simulink model "QPSK_system_v3e"  (R2012b)
settings: Solver=FixedStepDiscrete  SolverMode=SingleTasking  StartTime=0.0  StopTime=6000  FixedStep=1  RelTol=1e-3
libraries: simulink x30, dspsigops x2, dspbuff3 x1, dspsrcs4 x1
(part 1 of 4)
settings Model: FPTRunName=FPA_Reference  Creator=Carl  LastModifiedBy=castone
settings DataIOCC: SignalLogging=off
settings OptimizationCC: BlockReduction=off  ConditionallyExecuteInputs=off  InlineParams=on
settings DebuggingCC: AlgebraicLoopMsg=error
settings HardwareCC: ProdHWDeviceType=ASIC/FPGA->ASIC/FPGA  ProdEqTarget=off

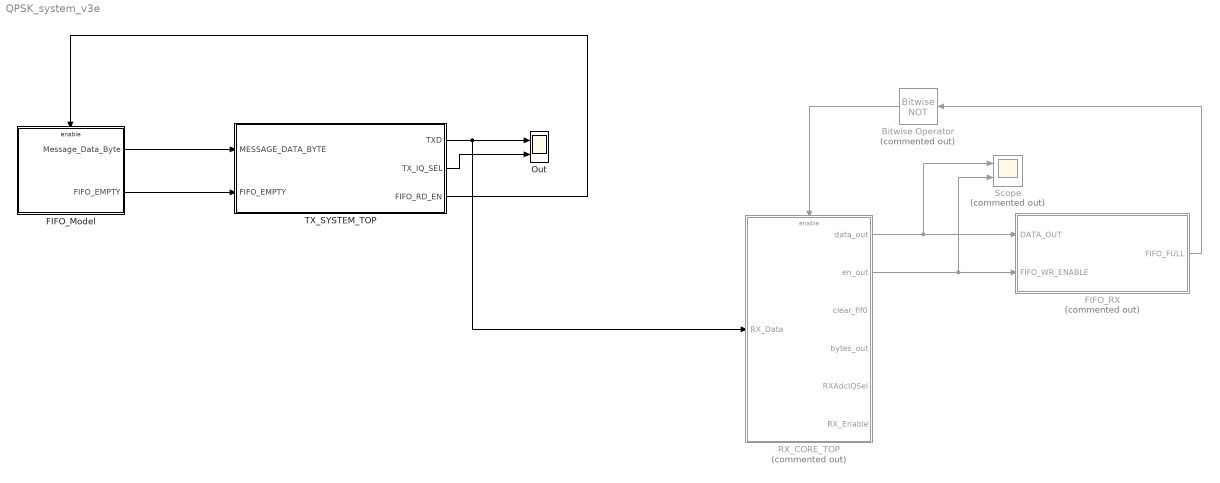
== system QPSK_system_v3e ==
  Bitwise Operator : simulink/Logic and Bit Operations/Bitwise Operator  Commented=on  logicop=NOT  UseBitMask=off  BitMask=bin2dec('11011001')  BitMaskRealWorld=Stored Integer
  FIFO_Model : Subsystem
  FIFO_RX : Subsystem  Commented=on
  Out : Scope  NumInputPorts=2
      settings: YMin=-5~-5  YMax=5~5  SaveName=ScopeData7
  RX_CORE_TOP : Subsystem  Commented=on
  Scope : Scope  Commented=on  NumInputPorts=2
      settings: YMin=-5~-5  YMax=5~5  SaveName=ScopeData20
  TX_SYSTEM_TOP : Subsystem
  wires:
  FIFO_Model/1(Message_Data_Byte) -> TX_SYSTEM_TOP/1(MESSAGE_DATA_BYTE)
  FIFO_Model/2(FIFO_EMPTY) -> TX_SYSTEM_TOP/2(FIFO_EMPTY)
  TX_SYSTEM_TOP/3(FIFO_RD_EN) -> FIFO_Model/Enable
  TX_SYSTEM_TOP/1(TXD) -> RX_CORE_TOP/1(RX_Data), Out/1
  TX_SYSTEM_TOP/2(TX_IQ_SEL) -> Out/2
  RX_CORE_TOP/1(data_out) -> FIFO_RX/1(DATA_OUT), Scope/1
  RX_CORE_TOP/2(en_out) -> FIFO_RX/2(FIFO_WR_ENABLE), Scope/2
  Bitwise Operator/1 -> RX_CORE_TOP/Enable
  FIFO_RX/1(FIFO_FULL) -> Bitwise Operator/1

== system QPSK_system_v3e/FIFO_Model ==
  Enable : EnablePort
  Compare To Constant5 : simulink/Logic and Bit Operations/Compare To Constant  relop===  const=17  OutDataTypeStr=boolean  ZeroCross=off
  Delay : Delay  DelayLength=1  InitialCondition=0
  Message_Data_LUT : LookupNDDirect  NumberOfTableDimensions=1  Table="[12        0        0        1        104        101        108        108        111        32        119        111        114        108        100        33        198        228]"  DiagnosticForOutOfRangeInput=Error  TableDataTypeStr=uint8
  Scope : Scope
  reset_counter : Subsystem  AncestorBlock=hdldemolib/HDL Streaming FFT/enable_counter
  Message_Data_Byte : Outport
  FIFO_EMPTY : Outport  Port=2
  wires:
  Message_Data_LUT/1 -> Message_Data_Byte/1
  reset_counter/1(sclock) -> Compare To Constant5/1, Scope/1, Message_Data_LUT/1
  Compare To Constant5/1 -> Delay/1, FIFO_EMPTY/1
  Delay/1 -> reset_counter/1(reset)

== system QPSK_system_v3e/FIFO_RX ==
  DATA_OUT : Inport
  FIFO_WR_ENABLE : Inport  Port=2
  Bitwise Operator : simulink/Logic and Bit Operations/Bitwise Operator  logicop=AND  UseBitMask=off  NumInputPorts=2  BitMask=bin2dec('11011001')  BitMaskRealWorld=Stored Integer
  Bitwise Operator1 : simulink/Logic and Bit Operations/Bitwise Operator  logicop=NOT  UseBitMask=off  BitMask=bin2dec('11011001')  BitMaskRealWorld=Stored Integer
  Data Type Conversion : DataTypeConversion  OutDataTypeStr=boolean
  Delay : Delay  InitialCondition=0
  Queue : dspbuff3/Queue  depth=18  trigger=Rising edge  overflow=Ignore  pes=Warning  eso=off  fso=on  nso=on  clr=off  clrOutport=off  adf=on
  print : Subsystem  TreatAsAtomicUnit=on
  FIFO_FULL : Outport
  wires:
  Queue/2 -> Delay/1
  Data Type Conversion/1 -> Queue/2, Bitwise Operator/1
  FIFO_WR_ENABLE/1 -> Data Type Conversion/1
  DATA_OUT/1 -> Queue/1, print/1(In1)
  Bitwise Operator1/1 -> Bitwise Operator/2
  Bitwise Operator/1 -> print/Enable
  Delay/1 -> FIFO_FULL/1, Bitwise Operator1/1

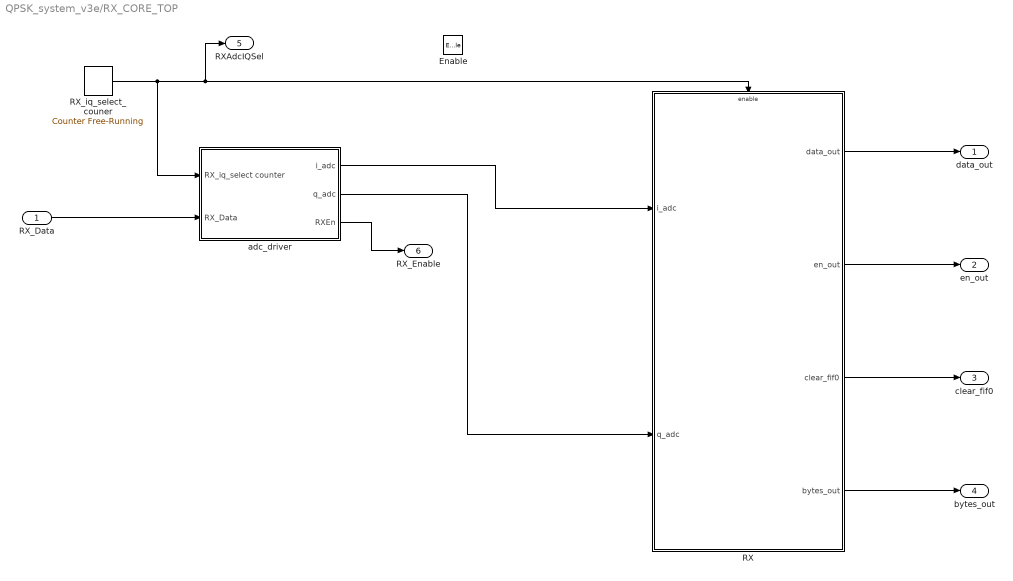
== system QPSK_system_v3e/RX_CORE_TOP ==
  RX_Data : Inport
  Enable : EnablePort
  RX : Subsystem
  RX_iq_select_couner : simulink/Sources/Counter Free-Running  NumBits=1  tsamp=-1
  adc_driver : Subsystem
  data_out : Outport
  en_out : Outport  Port=2
  clear_fif0 : Outport  Port=3
  bytes_out : Outport  Port=4
  RXAdcIQSel : Outport  Port=5
  RX_Enable : Outport  Port=6
  wires:
  RX/1(data_out) -> data_out/1
  RX/2(en_out) -> en_out/1
  RX/3(clear_fif0) -> clear_fif0/1
  RX/4(bytes_out) -> bytes_out/1
  RX_iq_select_couner/1 -> RX/Enable, RXAdcIQSel/1, adc_driver/1(RX_iq_select counter)
  adc_driver/3(RXEn) -> RX_Enable/1
  RX_Data/1 -> adc_driver/2(RX_Data)
  adc_driver/1(i_adc) -> RX/1(i_adc)
  adc_driver/2(q_adc) -> RX/2(q_adc)

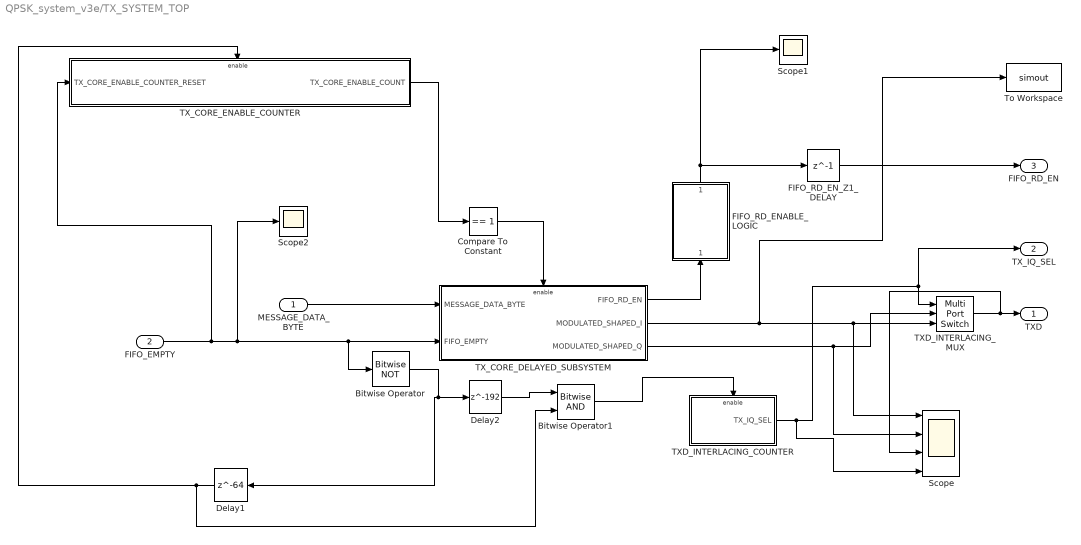
== system QPSK_system_v3e/TX_SYSTEM_TOP ==
  MESSAGE_DATA_BYTE : Inport
  FIFO_EMPTY : Inport  Port=2
  Bitwise Operator : simulink/Logic and Bit Operations/Bitwise Operator  logicop=NOT  UseBitMask=off  BitMask=bin2dec('11011001')  BitMaskRealWorld=Stored Integer
  Bitwise Operator1 : simulink/Logic and Bit Operations/Bitwise Operator  logicop=AND  UseBitMask=off  NumInputPorts=2  BitMask=bin2dec('11011001')  BitMaskRealWorld=Stored Integer
  Compare To Constant : simulink/Logic and Bit Operations/Compare To Constant  relop===  const=1  OutDataTypeStr=boolean
  Delay1 : Delay  DelayLength=64  InitialCondition=0
  Delay2 : Delay  DelayLength=192  InitialCondition=0
  FIFO_RD_ENABLE_LOGIC : Subsystem  AncestorBlock=hdldemolib/HDL Streaming FFT/enable_counter
  FIFO_RD_EN_Z1_DELAY : Delay  DelayLength=1  InitialCondition=0
  Scope : Scope  NumInputPorts=4
      settings: YMin=-5~-5~-5~-5  YMax=5~5~5~5
  Scope1 : Scope
      settings: SaveName=ScopeData8
  Scope2 : Scope
      settings: SaveName=ScopeData9
  "TXD_INTERLACING_COUNTER " : Subsystem
  TXD_INTERLACING_MUX : MultiPortSwitch  DataPortOrder=Zero-based contiguous  Inputs=2  zeroidx=on
  TX_CORE_DELAYED_SUBSYSTEM : Subsystem
  TX_CORE_ENABLE_COUNTER : Subsystem  AncestorBlock=hdldemolib/HDL Streaming FFT/enable_counter
  To Workspace : ToWorkspace  VariableName=simout  SampleTime=-1
  TXD : Outport
  TX_IQ_SEL : Outport  Port=2
  FIFO_RD_EN : Outport  Port=3
  wires:
  FIFO_RD_EN_Z1_DELAY/1 -> FIFO_RD_EN/1
  MESSAGE_DATA_BYTE/1 -> TX_CORE_DELAYED_SUBSYSTEM/1(MESSAGE_DATA_BYTE)
  TXD_INTERLACING_MUX/1 -> Scope/3, TXD/1
  TX_CORE_DELAYED_SUBSYSTEM/3(MODULATED_SHAPED_Q) -> Scope/2, TXD_INTERLACING_MUX/2
  TX_CORE_DELAYED_SUBSYSTEM/2(MODULATED_SHAPED_I) -> To Workspace/1, Scope/1, TXD_INTERLACING_MUX/3
  TX_CORE_ENABLE_COUNTER/1(TX_CORE_ENABLE_COUNT) -> Compare To Constant/1
  "TXD_INTERLACING_COUNTER "/1("TX_IQ_SEL ") -> Scope/4, TX_IQ_SEL/1, TXD_INTERLACING_MUX/1
  FIFO_EMPTY/1 -> TX_CORE_ENABLE_COUNTER/1(TX_CORE_ENABLE_COUNTER_RESET), Scope2/1, TX_CORE_DELAYED_SUBSYSTEM/2(FIFO_EMPTY), Bitwise Operator/1
  Compare To Constant/1 -> TX_CORE_DELAYED_SUBSYSTEM/Enable
  TX_CORE_DELAYED_SUBSYSTEM/1(FIFO_RD_EN) -> FIFO_RD_ENABLE_LOGIC/1(FIFO_RD_ENABLE_LOGIC_INPUT)
  FIFO_RD_ENABLE_LOGIC/1(FIFO_RD_ENABLE_LOGIC_OUTPUT) -> Scope1/1, FIFO_RD_EN_Z1_DELAY/1
  Bitwise Operator/1 -> Delay2/1, Delay1/1
  Delay1/1 -> Bitwise Operator1/2, TX_CORE_ENABLE_COUNTER/Enable
  Delay2/1 -> Bitwise Operator1/1
  Bitwise Operator1/1 -> "TXD_INTERLACING_COUNTER "/Enable

== system QPSK_system_v3e/FIFO_Model/reset_counter ==
  reset : Inport
  Compare To Constant3 : simulink/Logic and Bit Operations/Compare To Constant  relop=>=  const=18  OutDataTypeStr=boolean  ZeroCross=off
  Constant1 : Constant  OutDataTypeStr=int8  SampleTime=-1
  Constant2 : Constant  Value=17  OutDataTypeStr=int8  SampleTime=-1
  Logical Operator : Logic  Operator=OR  AllPortsSameDT=off  OutDataTypeStr=boolean
  Sum : Sum  AccumDataTypeStr=int8  RndMeth=Nearest  SaturateOnIntegerOverflow=on
  Switch1 : Switch  Criteria=u2 ~= 0
  Unit Delay : UnitDelay  SampleTime=-1
  sclock : Outport
  wires:
  Switch1/1 -> Sum/2, sclock/1
  Unit Delay/1 -> Compare To Constant3/1, Switch1/3
  Constant2/1 -> Switch1/1
  Sum/1 -> Unit Delay/1
  Constant1/1 -> Sum/1
  Compare To Constant3/1 -> Logical Operator/2
  reset/1 -> Logical Operator/1
  Logical Operator/1 -> Switch1/2

== system QPSK_system_v3e/FIFO_RX/print ==
  In1 : Inport
  Enable : EnablePort
  MATLAB Function : MATLAB Function  TreatAsAtomicUnit=on
  To Workspace2 : ToWorkspace  VariableName=fix_out  SampleTime=-1
  wires:
  In1/1 -> To Workspace2/1, MATLAB Function/1(byte_in)

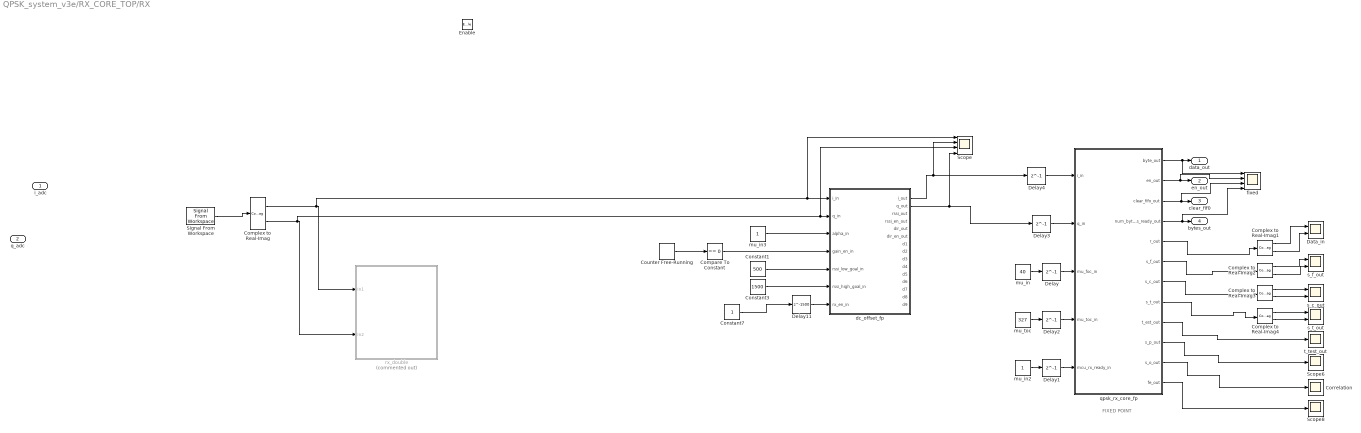
== system QPSK_system_v3e/RX_CORE_TOP/RX ==
  note: FIXED POINT
  i_adc : Inport
  q_adc : Inport  Port=2
  Enable : EnablePort
  Compare To Constant : simulink/Logic and Bit Operations/Compare To Constant  relop===  const=0  OutDataTypeStr=uint8
  Complex to Real-Imag{,1..4} (5 alike) : ComplexToRealImag
  Constant1 : Constant  Value=500  OutDataTypeStr=fixdt(0,24,0)  SampleTime=-1
  Constant3 : Constant  Value=1500  OutDataTypeStr=fixdt(0,24,0)  SampleTime=-1
  Constant7 : Constant  OutDataTypeStr=boolean  SampleTime=-1
  Correlation : Scope
      settings: SaveName=ScopeData11
  Counter Free-Running : simulink/Sources/Counter Free-Running  NumBits=16  tsamp=-1
  Data_in : Scope  NumInputPorts=2
      settings: YMin=-5~-5  YMax=5~5  SaveName=ScopeData17
  Delay{,1..4} (5 alike) : Delay  DelayLength=1  InitialCondition=0
  Delay11 : Delay  DelayLength=1500  InitialCondition=0
  Scope : Scope  NumInputPorts=4
      settings: YMin=-5~-5~-5~-5  YMax=5~5~5~5  SaveName=ScopeData21
  Scope6 : Scope
      settings: SaveName=ScopeData16
  Scope8 : Scope
      settings: SaveName=ScopeData18
  Signal From Workspace : dspsrcs4/Signal From Workspace  X=r  Ts=1  nsamps=1  OutputAfterFinalValue=Setting to zero  ignoreOrWarnInputAndFrameLengths=off
  dc_offset_fp : MATLAB Function  TreatAsAtomicUnit=on
  "fixed " : Scope  NumInputPorts=4
      settings: TimeRange=6000  YMin=0~-5~-5~-5  YMax=120~5~5~5  SaveName=ScopeData10
  mu_in : Constant  Value=40  OutDataTypeStr=fixdt(0,12,0)  SampleTime=-1
  mu_in2 : Constant  OutDataTypeStr=fixdt(0,1,0)  SampleTime=-1
  mu_in3 : Constant  OutDataTypeStr=fixdt(0,12,0)  SampleTime=-1
  mu_toc : Constant  Value=327  OutDataTypeStr=fixdt(0,12,0)  SampleTime=-1
  qpsk_rx_core_fp : MATLAB Function  TreatAsAtomicUnit=on
  rx_double : Subsystem  Commented=on
  s_c_out : Scope  NumInputPorts=2
      settings: YMin=-5~-5  YMax=5~5  SaveName=ScopeData13
  s_f_out : Scope  NumInputPorts=2
      settings: YMin=-5~-5  YMax=5~5  SaveName=ScopeData12
  s_t_out : Scope  NumInputPorts=2
      settings: YMin=-5~-5  YMax=5~5  SaveName=ScopeData14
  "t_test_out " : Scope
      settings: YMin=0  YMax=4.5  SaveName=ScopeData15
  data_out : Outport
  en_out : Outport  Port=2
  clear_fif0 : Outport  Port=3
  bytes_out : Outport  Port=4
  wires:
  qpsk_rx_core_fp/3(clear_fifo_out) -> "fixed "/3, clear_fif0/1
  qpsk_rx_core_fp/11(s_o_out) -> Correlation/1
  mu_toc/1 -> Delay2/1
  qpsk_rx_core_fp/4(num_bytes_ready_out) -> "fixed "/4, bytes_out/1
  qpsk_rx_core_fp/1(byte_out) -> "fixed "/1, data_out/1
  qpsk_rx_core_fp/2(en_out) -> "fixed "/2, en_out/1
  qpsk_rx_core_fp/5(r_out) -> Complex to Real-Imag1/1
  Complex to Real-Imag1/1 -> Data_in/1
  Complex to Real-Imag1/2 -> Data_in/2
  qpsk_rx_core_fp/6(s_f_out) -> Complex to Real-Imag2/1
  Complex to Real-Imag2/1 -> s_f_out/1
  Complex to Real-Imag2/2 -> s_f_out/2
  qpsk_rx_core_fp/7(s_c_out) -> Complex to Real-Imag3/1
  Complex to Real-Imag3/1 -> s_c_out/1
  Complex to Real-Imag3/2 -> s_c_out/2
  qpsk_rx_core_fp/8(s_t_out) -> Complex to Real-Imag4/1
  Complex to Real-Imag4/1 -> s_t_out/1
  Complex to Real-Imag4/2 -> s_t_out/2
  qpsk_rx_core_fp/9(t_est_out) -> "t_test_out "/1
  qpsk_rx_core_fp/10(s_p_out) -> Scope6/1
  qpsk_rx_core_fp/12(fe_out) -> Scope8/1
  mu_in2/1 -> Delay1/1
  dc_offset_fp/1(i_out) -> Scope/2, Delay4/1
  Constant1/1 -> dc_offset_fp/5(rssi_low_goal_in)
  Constant3/1 -> dc_offset_fp/6(rssi_high_goal_in)
  mu_in3/1 -> dc_offset_fp/3(alpha_in)
  Counter Free-Running/1 -> Compare To Constant/1
  Delay11/1 -> dc_offset_fp/7(rx_en_in)
  Constant7/1 -> Delay11/1
  dc_offset_fp/2(q_out) -> Scope/4, Delay3/1
  mu_in/1 -> Delay/1
  Delay4/1 -> qpsk_rx_core_fp/1(i_in)
  Delay3/1 -> qpsk_rx_core_fp/2(q_in)
  Delay/1 -> qpsk_rx_core_fp/3(mu_foc_in)
  Delay2/1 -> qpsk_rx_core_fp/4(mu_toc_in)
  Delay1/1 -> qpsk_rx_core_fp/5(mcu_rx_ready_in)
  Compare To Constant/1 -> dc_offset_fp/4(gain_en_in)
  Signal From Workspace/1 -> Complex to Real-Imag/1
  Complex to Real-Imag/1 -> Scope/1, dc_offset_fp/1(i_in), rx_double/1(In1)
  Complex to Real-Imag/2 -> Scope/3, dc_offset_fp/2(q_in), rx_double/2(In2)

== system QPSK_system_v3e/RX_CORE_TOP/adc_driver ==
  RX_iq_select counter : Inport
  RX_Data : Inport  Port=2
  Bitwise Operator : simulink/Logic and Bit Operations/Bitwise Operator  logicop=NOT  UseBitMask=off  BitMask=bin2dec('11011001')  BitMaskRealWorld=Stored Integer
  Constant : Constant  OutDataTypeStr=fixdt(0,1,0)  SampleTime=-1
  Sample and Hold : dspsigops/Sample and Hold  trig=Rising edge  initCond=0  latchinput=off
  Sample and Hold1 : dspsigops/Sample and Hold  trig=Rising edge  initCond=0  latchinput=off
  i_adc : Outport
  q_adc : Outport  Port=2
  RXEn : Outport  Port=3
  wires:
  RX_Data/1 -> Sample and Hold/1, Sample and Hold1/1
  Bitwise Operator/1 -> Sample and Hold1/Trigger
  Sample and Hold1/1 -> q_adc/1
  Sample and Hold/1 -> i_adc/1
  Constant/1 -> RXEn/1
  RX_iq_select counter/1 -> Bitwise Operator/1, Sample and Hold/Trigger

== system QPSK_system_v3e/TX_SYSTEM_TOP/FIFO_RD_ENABLE_LOGIC ==
  FIFO_RD_ENABLE_LOGIC_INPUT : Inport
  Bitwise Operator : simulink/Logic and Bit Operations/Bitwise Operator  logicop=AND  UseBitMask=off  NumInputPorts=2  BitMask=bin2dec('11011001')  BitMaskRealWorld=Stored Integer
  Compare To Constant : simulink/Logic and Bit Operations/Compare To Constant  relop===  const=1  OutDataTypeStr=boolean
  Compare To Constant1 : simulink/Logic and Bit Operations/Compare To Constant  relop===  const=0  OutDataTypeStr=boolean
  Delay : Delay  DelayLength=1  InitialCondition=0
  FIFO_RD_ENABLE_LOGIC_OUTPUT : Outport  InitialOutput=0
  wires:
  FIFO_RD_ENABLE_LOGIC_INPUT/1 -> Compare To Constant/1, Delay/1
  Delay/1 -> Compare To Constant1/1
  Compare To Constant/1 -> Bitwise Operator/1
  Compare To Constant1/1 -> Bitwise Operator/2
  Bitwise Operator/1 -> FIFO_RD_ENABLE_LOGIC_OUTPUT/1

== system QPSK_system_v3e/TX_SYSTEM_TOP/TXD_INTERLACING_COUNTER  ==
  Enable : EnablePort
  Counter Free-Running : simulink/Sources/Counter Free-Running  NumBits=1  tsamp=-1
  "TX_IQ_SEL " : Outport  InitialOutput=0
  wires:
  Counter Free-Running/1 -> "TX_IQ_SEL "/1

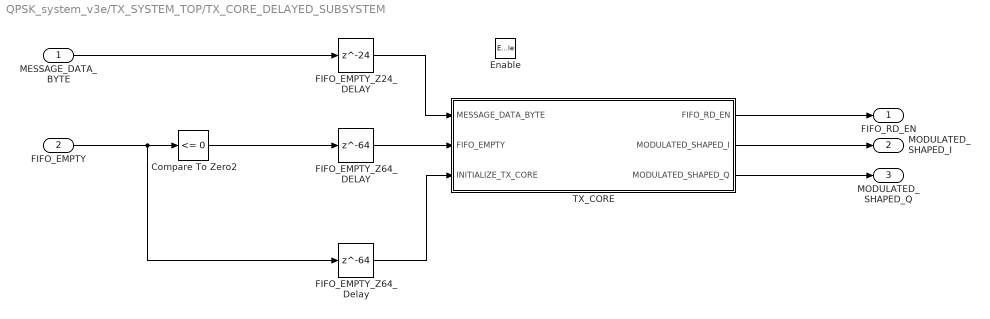
== system QPSK_system_v3e/TX_SYSTEM_TOP/TX_CORE_DELAYED_SUBSYSTEM ==
  MESSAGE_DATA_BYTE : Inport
  FIFO_EMPTY : Inport  Port=2
  Enable : EnablePort
  Compare To Zero2 : simulink/Logic and Bit Operations/Compare To Zero  relop=<=  OutDataTypeStr=boolean
  FIFO_EMPTY_Z24_DELAY : Delay  DelayLength=24  InitialCondition=0
  FIFO_EMPTY_Z64_DELAY : Delay  DelayLength=64  InitialCondition=0
  FIFO_EMPTY_Z64_Delay : Delay  DelayLength=64  InitialCondition=0
  TX_CORE : Subsystem
  FIFO_RD_EN : Outport  InitialOutput=0
  MODULATED_SHAPED_I : Outport  Port=2  InitialOutput=0
  MODULATED_SHAPED_Q : Outport  Port=3  InitialOutput=0
  wires:
  MESSAGE_DATA_BYTE/1 -> FIFO_EMPTY_Z24_DELAY/1
  FIFO_EMPTY_Z64_Delay/1 -> TX_CORE/3(INITIALIZE_TX_CORE)
  FIFO_EMPTY_Z64_DELAY/1 -> TX_CORE/2(FIFO_EMPTY)
  Compare To Zero2/1 -> FIFO_EMPTY_Z64_DELAY/1
  FIFO_EMPTY_Z24_DELAY/1 -> TX_CORE/1(MESSAGE_DATA_BYTE)
  TX_CORE/2(MODULATED_SHAPED_I) -> MODULATED_SHAPED_I/1
  TX_CORE/3(MODULATED_SHAPED_Q) -> MODULATED_SHAPED_Q/1
  FIFO_EMPTY/1 -> FIFO_EMPTY_Z64_Delay/1, Compare To Zero2/1
  TX_CORE/1(FIFO_RD_EN) -> FIFO_RD_EN/1

== system QPSK_system_v3e/TX_SYSTEM_TOP/TX_CORE_ENABLE_COUNTER ==
  TX_CORE_ENABLE_COUNTER_RESET : Inport
  Enable : EnablePort
  Compare To Constant : simulink/Logic and Bit Operations/Compare To Constant  relop===  const=1  OutDataTypeStr=boolean
  Constant1 : Constant  OutDataTypeStr=uint32
  Constant2 : Constant  Value=0  OutDataTypeStr=uint32
  Logical Operator : Logic  Operator=OR  AllPortsSameDT=off  OutDataTypeStr=boolean
  Sum : Sum  OutDataTypeStr=uint32  RndMeth=Nearest  SaturateOnIntegerOverflow=on
  Switch1 : Switch  Criteria=u2 ~= 0
  Unit Delay1 : UnitDelay  SampleTime=-1
  TX_CORE_ENABLE_COUNT : Outport  InitialOutput=0
  wires:
  Switch1/1 -> Unit Delay1/1
  Sum/1 -> Switch1/3
  Constant2/1 -> Switch1/1
  Constant1/1 -> Sum/1
  Logical Operator/1 -> Switch1/2
  Unit Delay1/1 -> TX_CORE_ENABLE_COUNT/1, Sum/2, Compare To Constant/1
  TX_CORE_ENABLE_COUNTER_RESET/1 -> Logical Operator/1
  Compare To Constant/1 -> Logical Operator/2

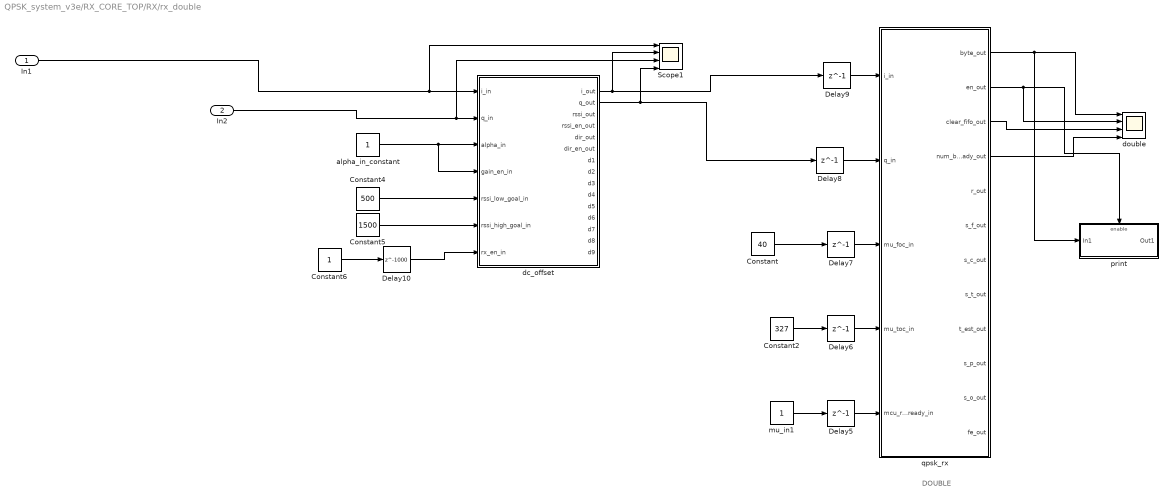
== system QPSK_system_v3e/RX_CORE_TOP/RX/rx_double ==
  note: DOUBLE
  In1 : Inport
  In2 : Inport  Port=2
  Constant : Constant  Value=40
  Constant2 : Constant  Value=327
  Constant4 : Constant  Value=500  OutDataTypeStr=double
  Constant5 : Constant  Value=1500  OutDataTypeStr=double
  Constant6 : Constant
  Delay10 : Delay  DelayLength=1000  InitialCondition=0
  Delay{5..9} (5 alike) : Delay  DelayLength=1  InitialCondition=0
  Scope1 : Scope  NumInputPorts=4
      settings: YMin=-5~-5~-5~-5  YMax=5~5~5~5  SaveName=ScopeData22
  alpha_in_constant : Constant  OutDataTypeStr=double  SampleTime=-1
  dc_offset : MATLAB Function  TreatAsAtomicUnit=on
  double : Scope  NumInputPorts=4
      settings: YMin=0~-5~-5~-5  YMax=120~5~5~5  SaveName=ScopeData19
  mu_in1 : Constant  OutDataTypeStr=fixdt(0,1,0)  SampleTime=-1
  print : Subsystem  TreatAsAtomicUnit=on
  qpsk_rx : MATLAB Function  TreatAsAtomicUnit=on
  wires:
  Constant6/1 -> Delay10/1
  Delay10/1 -> dc_offset/7(rx_en_in)
  In1/1 -> Scope1/1, dc_offset/1(i_in)
  dc_offset/1(i_out) -> Scope1/2, Delay9/1
  dc_offset/2(q_out) -> Scope1/4, Delay8/1
  Constant/1 -> Delay7/1
  qpsk_rx/3(clear_fifo_out) -> double/3
  Delay5/1 -> qpsk_rx/5(mcu_rx_ready_in)
  Constant4/1 -> dc_offset/5(rssi_low_goal_in)
  alpha_in_constant/1 -> dc_offset/4(gain_en_in), dc_offset/3(alpha_in)
  qpsk_rx/1(byte_out) -> double/1, print/1(In1)
  qpsk_rx/2(en_out) -> print/Enable, double/2
  Delay8/1 -> qpsk_rx/2(q_in)
  Constant2/1 -> Delay6/1
  mu_in1/1 -> Delay5/1
  Constant5/1 -> dc_offset/6(rssi_high_goal_in)
  qpsk_rx/4(num_bytes_ready_out) -> double/4
  Delay6/1 -> qpsk_rx/4(mu_toc_in)
  Delay7/1 -> qpsk_rx/3(mu_foc_in)
  Delay9/1 -> qpsk_rx/1(i_in)
  In2/1 -> Scope1/3, dc_offset/2(q_in)

== system QPSK_system_v3e/TX_SYSTEM_TOP/TX_CORE_DELAYED_SUBSYSTEM/TX_CORE ==
  MESSAGE_DATA_BYTE : Inport
  FIFO_EMPTY : Inport  Port=2
  INITIALIZE_TX_CORE : Inport  Port=3
  GEN_MOD_SHAPED_TX_DATA_PACKET : Subsystem
  FIFO_RD_EN : Outport
  MODULATED_SHAPED_I : Outport  Port=2
  MODULATED_SHAPED_Q : Outport  Port=3
  wires:
  INITIALIZE_TX_CORE/1 -> GEN_MOD_SHAPED_TX_DATA_PACKET/2(INITIALIZE_TX_CORE)
  GEN_MOD_SHAPED_TX_DATA_PACKET/2(MODULATED_SHAPED_I) -> MODULATED_SHAPED_I/1
  GEN_MOD_SHAPED_TX_DATA_PACKET/1(FIFO_RD_EN) -> FIFO_RD_EN/1
  MESSAGE_DATA_BYTE/1 -> GEN_MOD_SHAPED_TX_DATA_PACKET/1(MESSAGE_DATA_BYTE)
  GEN_MOD_SHAPED_TX_DATA_PACKET/3(MODULATED_SHAPED_Q) -> MODULATED_SHAPED_Q/1
  FIFO_EMPTY/1 -> GEN_MOD_SHAPED_TX_DATA_PACKET/Enable

== system QPSK_system_v3e/RX_CORE_TOP/RX/rx_double/print ==
  In1 : Inport
  Enable : EnablePort
  MATLAB Function : MATLAB Function  TreatAsAtomicUnit=on
  To Workspace1 : ToWorkspace  VariableName=double_out  SampleTime=-1
  Out1 : Outport
  wires:
  In1/1 -> To Workspace1/1, MATLAB Function/1(byte_in)
  ? -> Out1/1

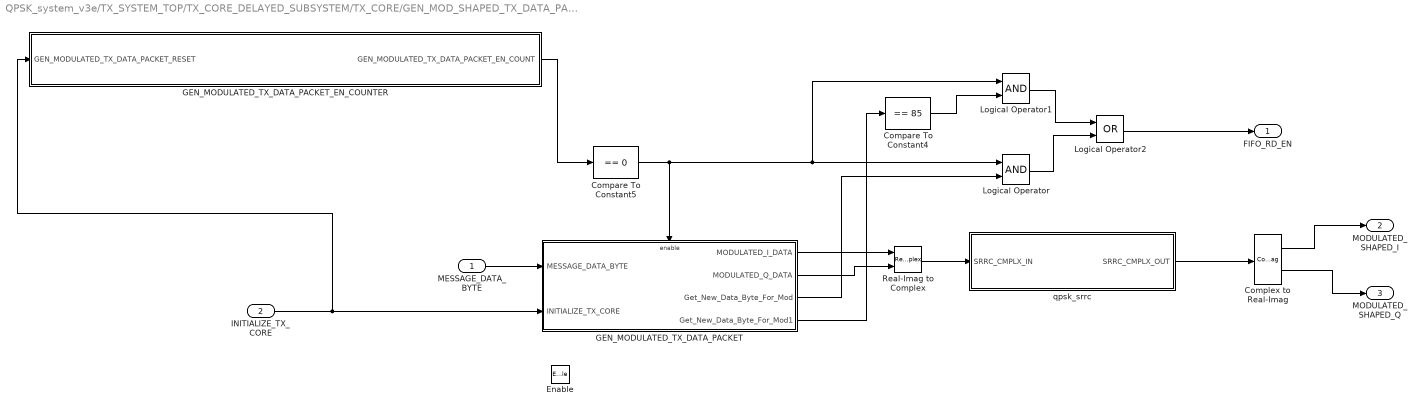
== system QPSK_system_v3e/TX_SYSTEM_TOP/TX_CORE_DELAYED_SUBSYSTEM/TX_CORE/GEN_MOD_SHAPED_TX_DATA_PACKET ==
  MESSAGE_DATA_BYTE : Inport
  INITIALIZE_TX_CORE : Inport  Port=2
  Enable : EnablePort
  Compare To Constant4 : simulink/Logic and Bit Operations/Compare To Constant  relop===  const=85  OutDataTypeStr=boolean  ZeroCross=off
  Compare To Constant5 : simulink/Logic and Bit Operations/Compare To Constant  relop===  const=0  OutDataTypeStr=boolean  ZeroCross=off
  Complex to Real-Imag : ComplexToRealImag
  GEN_MODULATED_TX_DATA_PACKET : Subsystem
  GEN_MODULATED_TX_DATA_PACKET_EN_COUNTER : Subsystem  AncestorBlock=hdldemolib/HDL Streaming FFT/enable_counter
  Logical Operator : Logic  AllPortsSameDT=off  OutDataTypeStr=boolean
  Logical Operator1 : Logic  AllPortsSameDT=off  OutDataTypeStr=boolean
  Logical Operator2 : Logic  Operator=OR  AllPortsSameDT=off  OutDataTypeStr=boolean
  Real-Imag to Complex : RealImagToComplex
  "qpsk_srrc " : Subsystem
  FIFO_RD_EN : Outport  InitialOutput=0
  MODULATED_SHAPED_I : Outport  Port=2  InitialOutput=0
  MODULATED_SHAPED_Q : Outport  Port=3  InitialOutput=0
  wires:
  Complex to Real-Imag/1 -> MODULATED_SHAPED_I/1
  Complex to Real-Imag/2 -> MODULATED_SHAPED_Q/1
  GEN_MODULATED_TX_DATA_PACKET/1(MODULATED_I_DATA) -> Real-Imag to Complex/1
  GEN_MODULATED_TX_DATA_PACKET/2(MODULATED_Q_DATA) -> Real-Imag to Complex/2
  MESSAGE_DATA_BYTE/1 -> GEN_MODULATED_TX_DATA_PACKET/1(MESSAGE_DATA_BYTE)
  GEN_MODULATED_TX_DATA_PACKET/3(Get_New_Data_Byte_For_Mod) -> Logical Operator/2
  Compare To Constant5/1 -> Logical Operator1/1, Logical Operator/1, GEN_MODULATED_TX_DATA_PACKET/Enable
  Compare To Constant4/1 -> Logical Operator1/2
  GEN_MODULATED_TX_DATA_PACKET/4(Get_New_Data_Byte_For_Mod1) -> Compare To Constant4/1
  Logical Operator/1 -> Logical Operator2/2
  Logical Operator1/1 -> Logical Operator2/1
  Logical Operator2/1 -> FIFO_RD_EN/1
  GEN_MODULATED_TX_DATA_PACKET_EN_COUNTER/1(GEN_MODULATED_TX_DATA_PACKET_EN_COUNT) -> Compare To Constant5/1
  INITIALIZE_TX_CORE/1 -> GEN_MODULATED_TX_DATA_PACKET_EN_COUNTER/1(GEN_MODULATED_TX_DATA_PACKET_RESET), GEN_MODULATED_TX_DATA_PACKET/2(INITIALIZE_TX_CORE)
  Real-Imag to Complex/1 -> "qpsk_srrc "/1(SRRC_CMPLX_IN)
  "qpsk_srrc "/1(SRRC_CMPLX_OUT) -> Complex to Real-Imag/1

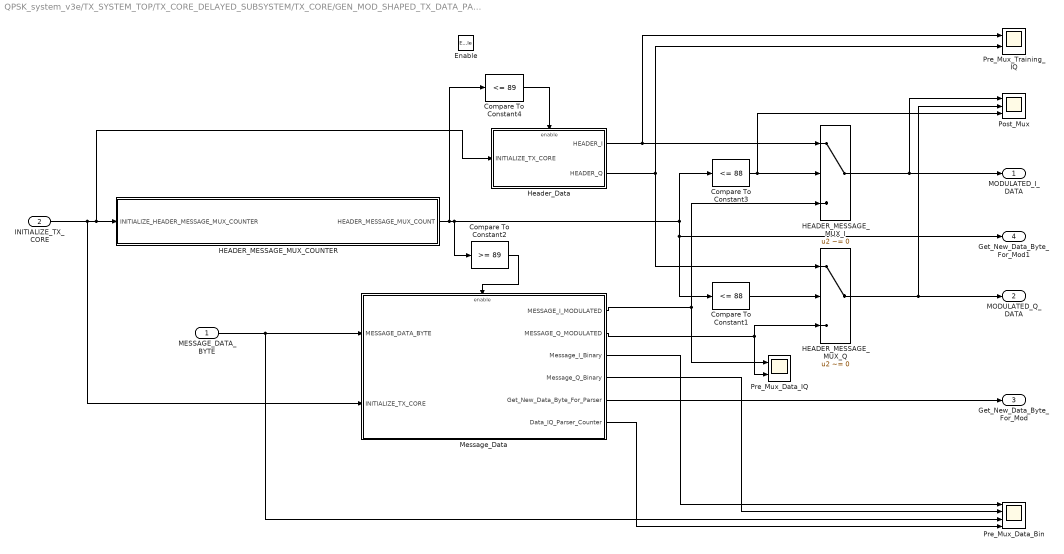
== system QPSK_system_v3e/TX_SYSTEM_TOP/TX_CORE_DELAYED_SUBSYSTEM/TX_CORE/GEN_MOD_SHAPED_TX_DATA_PACKET/GEN_MODULATED_TX_DATA_PACKET ==
  MESSAGE_DATA_BYTE : Inport
  INITIALIZE_TX_CORE : Inport  Port=2
  Enable : EnablePort
  Compare To Constant1 : simulink/Logic and Bit Operations/Compare To Constant  relop=<=  const=88  OutDataTypeStr=boolean  ZeroCross=off
  Compare To Constant2 : simulink/Logic and Bit Operations/Compare To Constant  relop=>=  const=89  OutDataTypeStr=boolean  ZeroCross=off
  Compare To Constant3 : simulink/Logic and Bit Operations/Compare To Constant  relop=<=  const=88  OutDataTypeStr=boolean  ZeroCross=off
  Compare To Constant4 : simulink/Logic and Bit Operations/Compare To Constant  relop=<=  const=89  OutDataTypeStr=boolean  ZeroCross=off
  HEADER_MESSAGE_MUX_COUNTER : Subsystem  AncestorBlock=hdldemolib/HDL Streaming FFT/enable_counter
  HEADER_MESSAGE_MUX_I : Switch  Criteria=u2 ~= 0  OutDataTypeStr=int8
  HEADER_MESSAGE_MUX_Q : Switch  Criteria=u2 ~= 0  OutDataTypeStr=int8
  Header_Data : Subsystem
  Message_Data : Subsystem
  Post_Mux : Scope  NumInputPorts=3
      settings: YMin=-5~-5~-5  YMax=5~5~5  SaveName=ScopeData2
  Pre_Mux_Data_Bin : Scope  NumInputPorts=4
      settings: TimeRange=1500  YMin=-0.2~-0.2~-10~-5  YMax=1.2~1.2~265~5  SaveName=ScopeData6
  Pre_Mux_Data_IQ : Scope  NumInputPorts=2
      settings: YMin=-5~-5  YMax=5~5  SaveName=ScopeData5
  Pre_Mux_Training_IQ : Scope  NumInputPorts=2
      settings: YMin=-5~-5  YMax=5~5  SaveName=ScopeData4
  MODULATED_I_DATA : Outport  InitialOutput=0
  MODULATED_Q_DATA : Outport  Port=2  InitialOutput=0
  Get_New_Data_Byte_For_Mod : Outport  Port=3  InitialOutput=0
  Get_New_Data_Byte_For_Mod1 : Outport  Port=4  InitialOutput=0
  wires:
  HEADER_MESSAGE_MUX_COUNTER/1(HEADER_MESSAGE_MUX_COUNT) -> Compare To Constant4/1, Compare To Constant3/1, Get_New_Data_Byte_For_Mod1/1, Compare To Constant1/1, Compare To Constant2/1
  HEADER_MESSAGE_MUX_I/1 -> MODULATED_I_DATA/1, Post_Mux/1
  Header_Data/1(HEADER_I) -> HEADER_MESSAGE_MUX_I/1, Pre_Mux_Training_IQ/1
  Compare To Constant1/1 -> HEADER_MESSAGE_MUX_Q/2
  HEADER_MESSAGE_MUX_Q/1 -> Post_Mux/2, MODULATED_Q_DATA/1
  Header_Data/2(HEADER_Q) -> HEADER_MESSAGE_MUX_Q/1, Pre_Mux_Training_IQ/2
  Message_Data/2(MESSAGE_Q_MODULATED) -> Pre_Mux_Data_IQ/2, HEADER_MESSAGE_MUX_Q/3
  Message_Data/1(MESSAGE_I_MODULATED) -> Pre_Mux_Data_IQ/1, HEADER_MESSAGE_MUX_I/3
  Message_Data/3(Message_I_Binary) -> Pre_Mux_Data_Bin/1
  Message_Data/4(Message_Q_Binary) -> Pre_Mux_Data_Bin/2
  Compare To Constant2/1 -> Message_Data/Enable
  Compare To Constant4/1 -> Header_Data/Enable
  MESSAGE_DATA_BYTE/1 -> Message_Data/1(MESSAGE_DATA_BYTE), Pre_Mux_Data_Bin/3
  Compare To Constant3/1 -> Post_Mux/3, HEADER_MESSAGE_MUX_I/2
  Message_Data/5(Get_New_Data_Byte_For_Parser) -> Get_New_Data_Byte_For_Mod/1
  Message_Data/6(Data_IQ_Parser_Counter) -> Pre_Mux_Data_Bin/4
  INITIALIZE_TX_CORE/1 -> HEADER_MESSAGE_MUX_COUNTER/1(INITIALIZE_HEADER_MESSAGE_MUX_COUNTER), Header_Data/1(INITIALIZE_TX_CORE), Message_Data/2(INITIALIZE_TX_CORE)

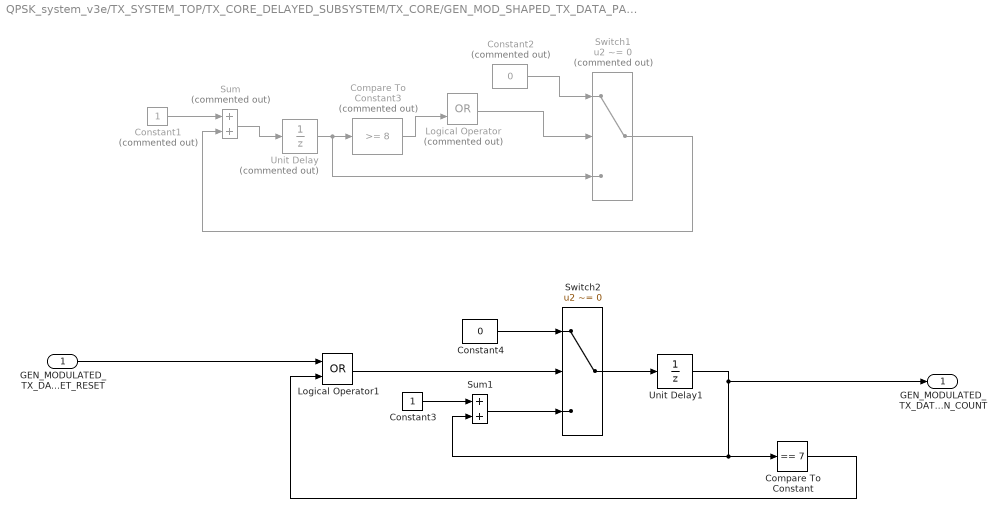
== system QPSK_system_v3e/TX_SYSTEM_TOP/TX_CORE_DELAYED_SUBSYSTEM/TX_CORE/GEN_MOD_SHAPED_TX_DATA_PACKET/GEN_MODULATED_TX_DATA_PACKET_EN_COUNTER ==
  GEN_MODULATED_TX_DATA_PACKET_RESET : Inport
  Compare To Constant3 : simulink/Logic and Bit Operations/Compare To Constant  Commented=on  relop=>=  const=8  OutDataTypeStr=boolean  ZeroCross=off
  Compare To Constant : simulink/Logic and Bit Operations/Compare To Constant  relop===  const=7  OutDataTypeStr=boolean
  Constant1 : Constant  Commented=on  OutDataTypeStr=int8  SampleTime=-1
  Constant2 : Constant  Commented=on  Value=0  OutDataTypeStr=int8  SampleTime=-1
  Constant3 : Constant  OutDataTypeStr=uint32
  Constant4 : Constant  Value=0  OutDataTypeStr=uint32
  Logical Operator : Logic  Commented=on  Operator=OR  AllPortsSameDT=off  OutDataTypeStr=boolean
  Logical Operator1 : Logic  Operator=OR  AllPortsSameDT=off  OutDataTypeStr=boolean
  Sum : Sum  Commented=on  OutDataTypeStr=int8  RndMeth=Nearest  SaturateOnIntegerOverflow=on
  Sum1 : Sum  OutDataTypeStr=uint32  RndMeth=Nearest  SaturateOnIntegerOverflow=on
  Switch1 : Switch  Commented=on  Criteria=u2 ~= 0
  Switch2 : Switch  Criteria=u2 ~= 0
  Unit Delay : UnitDelay  Commented=on  SampleTime=-1
  Unit Delay1 : UnitDelay  SampleTime=-1
  GEN_MODULATED_TX_DATA_PACKET_EN_COUNT : Outport  InitialOutput=0
  wires:
  Switch1/1 -> Sum/2
  Unit Delay/1 -> Compare To Constant3/1, Switch1/3
  Constant2/1 -> Switch1/1
  Sum/1 -> Unit Delay/1
  Constant1/1 -> Sum/1
  Compare To Constant3/1 -> Logical Operator/2
  Logical Operator/1 -> Switch1/2
  Switch2/1 -> Unit Delay1/1
  Sum1/1 -> Switch2/3
  Constant4/1 -> Switch2/1
  Constant3/1 -> Sum1/1
  Logical Operator1/1 -> Switch2/2
  Unit Delay1/1 -> GEN_MODULATED_TX_DATA_PACKET_EN_COUNT/1, Sum1/2, Compare To Constant/1
  Compare To Constant/1 -> Logical Operator1/2
  GEN_MODULATED_TX_DATA_PACKET_RESET/1 -> Logical Operator1/1

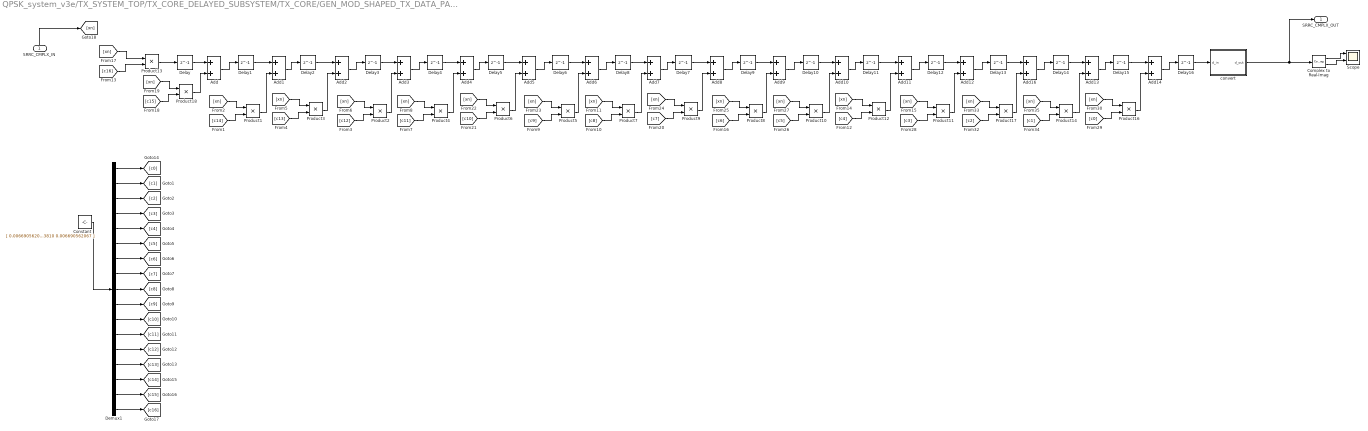
== system QPSK_system_v3e/TX_SYSTEM_TOP/TX_CORE_DELAYED_SUBSYSTEM/TX_CORE/GEN_MOD_SHAPED_TX_DATA_PACKET/qpsk_srrc  ==
  SRRC_CMPLX_IN : Inport
  Add{,1..14,16} (16 alike) : Sum
  Complex to Real-Imag : ComplexToRealImag
  Constant : Constant  Value=|  OutDataTypeStr=fixdt(1,12,11)
      | [
      | 0.006690562067
      | -0.005768593810
      | -0.011827354519
      | 0.020586915021
      | 0.016726405168
      | -0.053692342207
      | -0.020253031546
      | 0.196043589067
      | 0.336822413190
      | 0.196043589067
      | -0.020253031546
      | -0.053692342207
      | 0.016726405168
      | 0.020586915021
      | -0.011827354519
      | -0.005768593810
      | 0.006690562067
      | ]
  Delay{,1..16} (17 alike) : Delay  DelayLength=1  InitialCondition=0
  Demux1 : Demux  Outputs=17
  Product{1..14,16..18} (17 alike) : Product  RndMeth=Zero
  Scope : Scope  NumInputPorts=2
      settings: YMin=-5~-5  YMax=5~5  SaveName=ScopeData23
  convert : MATLAB Function  TreatAsAtomicUnit=on
  SRRC_CMPLX_OUT : Outport
  wires:
  convert/1(d_out) -> SRRC_CMPLX_OUT/1, Complex to Real-Imag/1
  Complex to Real-Imag/1 -> Scope/1
  Complex to Real-Imag/2 -> Scope/2
  Constant/1 -> Demux1/1
  Demux1/2 -> [c1]
  Demux1/3 -> [c2]
  Demux1/4 -> [c3]
  Demux1/5 -> [c4]
  Demux1/6 -> [c5]
  Demux1/7 -> [c6]
  Demux1/8 -> [c7]
  Demux1/9 -> [c8]
  Demux1/10 -> [c9]
  Demux1/11 -> [c10]
  Demux1/12 -> [c11]
  Demux1/13 -> [c12]
  Demux1/14 -> [c13]
  Demux1/15 -> [c14]
  Demux1/16 -> [c15]
  Demux1/17 -> [c16]
  Demux1/1 -> [c0]
  Delay/1 -> Add/1
  Add/1 -> Delay1/1
  Product18/1 -> Add/2
  [c16] -> Product13/2
  Product13/1 -> Delay/1
  [xn] -> Product13/1
  [xn] -> Product18/1
  [c15] -> Product18/2
  Add1/1 -> Delay2/1
  Product1/1 -> Add1/2
  [xn] -> Product1/1
  [c14] -> Product1/2
  Delay1/1 -> Add1/1
  Add2/1 -> Delay3/1
  Product3/1 -> Add2/2
  [xn] -> Product3/1
  [c13] -> Product3/2
  Add3/1 -> Delay4/1
  Product2/1 -> Add3/2
  [xn] -> Product2/1
  [c12] -> Product2/2
  Delay3/1 -> Add3/1
  Delay2/1 -> Add2/1
  Add4/1 -> Delay5/1
  Product4/1 -> Add4/2
  [xn] -> Product4/1
  [c11] -> Product4/2
  Add5/1 -> Delay6/1
  Product6/1 -> Add5/2
  [xn] -> Product6/1
  [c10] -> Product6/2
  Add6/1 -> Delay8/1
  Product5/1 -> Add6/2
  [xn] -> Product5/1
  [c9] -> Product5/2
  Delay6/1 -> Add6/1
  Delay5/1 -> Add5/1
  Delay4/1 -> Add4/1
  Add7/1 -> Delay7/1
  Product7/1 -> Add7/2
  [xn] -> Product7/1
  [c8] -> Product7/2
  Add8/1 -> Delay9/1
  Product9/1 -> Add8/2
  [xn] -> Product9/1
  [c7] -> Product9/2
  Add9/1 -> Delay10/1
  Product8/1 -> Add9/2
  [xn] -> Product8/1
  [c6] -> Product8/2
  Delay9/1 -> Add9/1
  Delay7/1 -> Add8/1
  Add10/1 -> Delay11/1
  Product10/1 -> Add10/2
  [xn] -> Product10/1
  [c5] -> Product10/2
  Add11/1 -> Delay12/1
  Product12/1 -> Add11/2
  [xn] -> Product12/1
  [c4] -> Product12/2
  Add12/1 -> Delay13/1
  Product11/1 -> Add12/2
  [xn] -> Product11/1
  [c3] -> Product11/2
  Delay12/1 -> Add12/1
  Delay11/1 -> Add11/1
  Delay10/1 -> Add10/1
  Delay8/1 -> Add7/1
  Add16/1 -> Delay14/1
  Product17/1 -> Add16/2
  [xn] -> Product17/1
  [c2] -> Product17/2
  Add13/1 -> Delay15/1
  Product14/1 -> Add13/2
  [xn] -> Product14/1
  [c1] -> Product14/2
  Add14/1 -> Delay16/1
  Product16/1 -> Add14/2
  [xn] -> Product16/1
  [c0] -> Product16/2
  Delay15/1 -> Add14/1
  Delay14/1 -> Add13/1
  Delay13/1 -> Add16/1
  SRRC_CMPLX_IN/1 -> [xn]
  Delay16/1 -> convert/1(d_in)

== system QPSK_system_v3e/TX_SYSTEM_TOP/TX_CORE_DELAYED_SUBSYSTEM/TX_CORE/GEN_MOD_SHAPED_TX_DATA_PACKET/GEN_MODULATED_TX_DATA_PACKET/HEADER_MESSAGE_MUX_COUNTER ==
  INITIALIZE_HEADER_MESSAGE_MUX_COUNTER : Inport
  Compare To Constant3 : simulink/Logic and Bit Operations/Compare To Constant  relop=>=  const=1024  OutDataTypeStr=boolean  ZeroCross=off
  Constant1 : Constant  OutDataTypeStr=int8  SampleTime=-1
  Constant2 : Constant  Value=0  OutDataTypeStr=int8  SampleTime=-1
  Logical Operator : Logic  Operator=OR  AllPortsSameDT=off  OutDataTypeStr=boolean
  Sum : Sum  OutDataTypeStr=uint32  RndMeth=Nearest  SaturateOnIntegerOverflow=on
  Switch1 : Switch  Criteria=u2 ~= 0
  Unit Delay : UnitDelay  SampleTime=-1
  HEADER_MESSAGE_MUX_COUNT : Outport
  wires:
  Switch1/1 -> Sum/2, HEADER_MESSAGE_MUX_COUNT/1
  Unit Delay/1 -> Compare To Constant3/1, Switch1/3
  Constant2/1 -> Switch1/1
  Sum/1 -> Unit Delay/1
  Constant1/1 -> Sum/1
  Compare To Constant3/1 -> Logical Operator/2
  INITIALIZE_HEADER_MESSAGE_MUX_COUNTER/1 -> Logical Operator/1
  Logical Operator/1 -> Switch1/2

== system QPSK_system_v3e/TX_SYSTEM_TOP/TX_CORE_DELAYED_SUBSYSTEM/TX_CORE/GEN_MOD_SHAPED_TX_DATA_PACKET/GEN_MODULATED_TX_DATA_PACKET/Header_Data ==
  INITIALIZE_TX_CORE : Inport
  Enable : EnablePort
  HEADER_SYMBOL_COUNTER : Subsystem  AncestorBlock=hdldemolib/HDL Streaming FFT/enable_counter
  Pad_Training_LUT_I : LookupNDDirect  NumberOfTableDimensions=1  Table=|  DiagnosticForOutOfRangeInput=Error  TableDataTypeStr=int8
      | [1
      | -1
      | 1
      | -1
      | 1
      | -1
      | 1
      | -1
      | 1
      | -1
      | 1
      | -1
      | 1
      | -1
      | 1
      | -1
      | 1
      | -1
      | 1
      | -1
      | 1
      | -1
      | 1
      | -1
      | 1
      | 1
      | -1
      | -1
      | 1
      | 1
      | -1
      | -1
      | 1
      | -1
      | -1
      | -1
      | -1
      | 1
      | -1
      | 1
      | 1
      | -1
      | -1
      | 1
      | 1
      | 1
      | -1
      | 1
      | 1
      | 1
      | -1
      | 1
      | -1
      | 1
      | 1
      | 1
      | -1
      | 1
      | 1
      | 1
      | 1
      | -1
      | 1
      | 1
      | -1
      | -1
      | -1
      | -1
      | 1
      | 1
      | 1
      | -1
      | -1
      | -1
      | 1
      | 1
      | 1
      | 1
      | -1
      | 1
      | 1
      | 1
      | 1
      | 1
      | -1
      | -1
      | -1
      | 1
      | 1
      | ]
  Pad_Training_LUT_Q : LookupNDDirect  NumberOfTableDimensions=1  Table=|  DiagnosticForOutOfRangeInput=Error  TableDataTypeStr=int8
      | [1
      | -1
      | 1
      | -1
      | 1
      | -1
      | 1
      | -1
      | 1
      | -1
      | 1
      | -1
      | 1
      | -1
      | 1
      | -1
      | 1
      | -1
      | 1
      | -1
      | 1
      | -1
      | 1
      | -1
      | 1
      | -1
      | 1
      | 1
      | 1
      | -1
      | -1
      | -1
      | -1
      | 1
      | 1
      | -1
      | 1
      | 1
      | -1
      | -1
      | -1
      | 1
      | -1
      | -1
      | 1
      | 1
      | 1
      | -1
      | -1
      | 1
      | 1
      | 1
      | -1
      | -1
      | -1
      | -1
      | -1
      | -1
      | 1
      | 1
      | -1
      | 1
      | -1
      | 1
      | 1
      | -1
      | -1
      | 1
      | -1
      | -1
      | 1
      | 1
      | -1
      | -1
      | -1
      | -1
      | -1
      | 1
      | 1
      | 1
      | 1
      | -1
      | -1
      | -1
      | -1
      | 1
      | -1
      | 1
      | -1
      | ]
  Training Counter : Scope  NumInputPorts=2
      settings: YMin=-5~-5  YMax=5~5  SaveName=ScopeData3
  HEADER_I : Outport  InitialOutput=0
  HEADER_Q : Outport  Port=2  InitialOutput=0
  wires:
  Pad_Training_LUT_I/1 -> HEADER_I/1
  HEADER_SYMBOL_COUNTER/1(HEADER_SYMBOL_COUNT) -> Training Counter/1, Pad_Training_LUT_I/1, Pad_Training_LUT_Q/1
  Pad_Training_LUT_Q/1 -> HEADER_Q/1
  INITIALIZE_TX_CORE/1 -> HEADER_SYMBOL_COUNTER/1(INITIALIZE_HEADER_SYMBOL_COUNTER), Training Counter/2

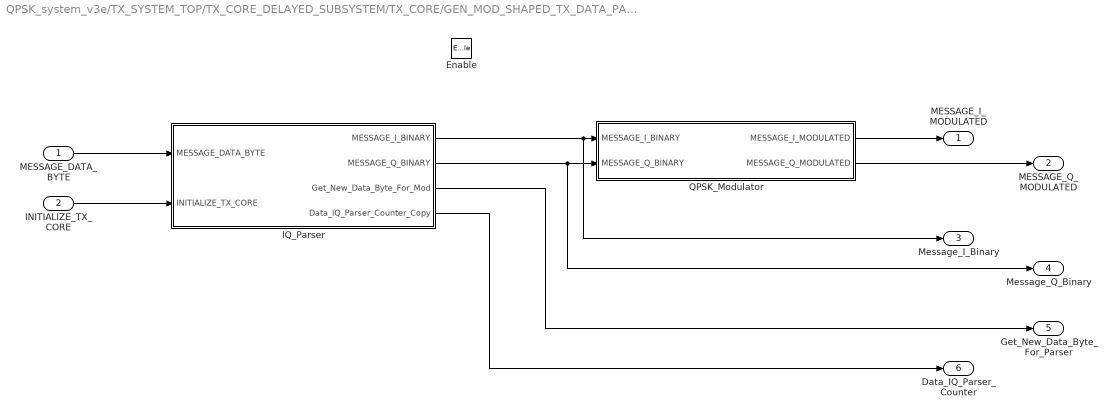
== system QPSK_system_v3e/TX_SYSTEM_TOP/TX_CORE_DELAYED_SUBSYSTEM/TX_CORE/GEN_MOD_SHAPED_TX_DATA_PACKET/GEN_MODULATED_TX_DATA_PACKET/Message_Data ==
  MESSAGE_DATA_BYTE : Inport
  INITIALIZE_TX_CORE : Inport  Port=2
  Enable : EnablePort
  IQ_Parser : Subsystem
  QPSK_Modulator : Subsystem
  MESSAGE_I_MODULATED : Outport  InitialOutput=0
  MESSAGE_Q_MODULATED : Outport  Port=2  InitialOutput=0
  Message_I_Binary : Outport  Port=3  InitialOutput=0
  Message_Q_Binary : Outport  Port=4  InitialOutput=0
  Get_New_Data_Byte_For_Parser : Outport  Port=5  InitialOutput=0
  Data_IQ_Parser_Counter : Outport  Port=6  InitialOutput=0
  wires:
  IQ_Parser/1(MESSAGE_I_BINARY) -> Message_I_Binary/1, QPSK_Modulator/1(MESSAGE_I_BINARY)
  IQ_Parser/2(MESSAGE_Q_BINARY) -> Message_Q_Binary/1, QPSK_Modulator/2(MESSAGE_Q_BINARY)
  QPSK_Modulator/1(MESSAGE_I_MODULATED) -> MESSAGE_I_MODULATED/1
  QPSK_Modulator/2(MESSAGE_Q_MODULATED) -> MESSAGE_Q_MODULATED/1
  MESSAGE_DATA_BYTE/1 -> IQ_Parser/1(MESSAGE_DATA_BYTE)
  IQ_Parser/3(Get_New_Data_Byte_For_Mod) -> Get_New_Data_Byte_For_Parser/1
  IQ_Parser/4(Data_IQ_Parser_Counter_Copy) -> Data_IQ_Parser_Counter/1
  INITIALIZE_TX_CORE/1 -> IQ_Parser/2(INITIALIZE_TX_CORE)

== system QPSK_system_v3e/TX_SYSTEM_TOP/TX_CORE_DELAYED_SUBSYSTEM/TX_CORE/GEN_MOD_SHAPED_TX_DATA_PACKET/GEN_MODULATED_TX_DATA_PACKET/Header_Data/HEADER_SYMBOL_COUNTER ==
  INITIALIZE_HEADER_SYMBOL_COUNTER : Inport
  Compare To Constant : simulink/Logic and Bit Operations/Compare To Constant  relop===  const=88  OutDataTypeStr=boolean
  Constant1 : Constant  OutDataTypeStr=uint32
  Constant2 : Constant  Value=0  OutDataTypeStr=uint32
  Logical Operator : Logic  Operator=OR  AllPortsSameDT=off  OutDataTypeStr=boolean
  Sum : Sum  OutDataTypeStr=uint32  RndMeth=Nearest  SaturateOnIntegerOverflow=on
  Switch1 : Switch  Criteria=u2 ~= 0
  Unit Delay1 : UnitDelay  SampleTime=-1
  HEADER_SYMBOL_COUNT : Outport
  wires:
  Switch1/1 -> Unit Delay1/1
  Sum/1 -> Switch1/3
  Constant2/1 -> Switch1/1
  Constant1/1 -> Sum/1
  Logical Operator/1 -> Switch1/2
  Unit Delay1/1 -> HEADER_SYMBOL_COUNT/1, Sum/2, Compare To Constant/1
  INITIALIZE_HEADER_SYMBOL_COUNTER/1 -> Logical Operator/1
  Compare To Constant/1 -> Logical Operator/2

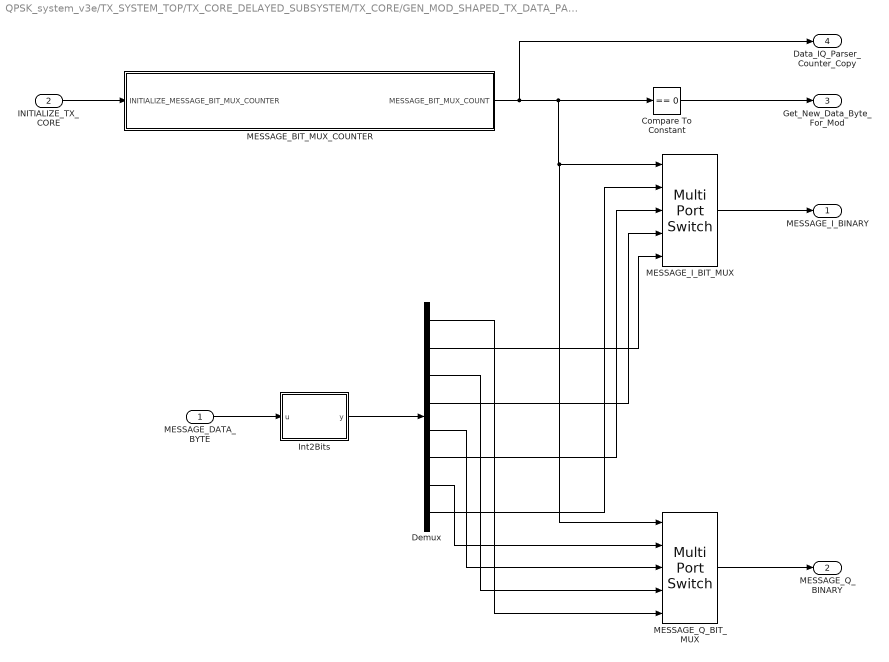
== system QPSK_system_v3e/TX_SYSTEM_TOP/TX_CORE_DELAYED_SUBSYSTEM/TX_CORE/GEN_MOD_SHAPED_TX_DATA_PACKET/GEN_MODULATED_TX_DATA_PACKET/Message_Data/IQ_Parser ==
  MESSAGE_DATA_BYTE : Inport
  INITIALIZE_TX_CORE : Inport  Port=2
  Compare To Constant : simulink/Logic and Bit Operations/Compare To Constant  relop===  const=0  OutDataTypeStr=boolean
  Demux : Demux  Outputs=8
  Int2Bits : MATLAB Function  TreatAsAtomicUnit=on
  MESSAGE_BIT_MUX_COUNTER : Subsystem  AncestorBlock=hdldemolib/HDL Streaming FFT/enable_counter
  MESSAGE_I_BIT_MUX : MultiPortSwitch  DataPortOrder=Zero-based contiguous  Inputs=4  zeroidx=on
  MESSAGE_Q_BIT_MUX : MultiPortSwitch  DataPortOrder=Zero-based contiguous  Inputs=4  zeroidx=on
  MESSAGE_I_BINARY : Outport
  MESSAGE_Q_BINARY : Outport  Port=2
  Get_New_Data_Byte_For_Mod : Outport  Port=3
  Data_IQ_Parser_Counter_Copy : Outport  Port=4
  wires:
  MESSAGE_Q_BIT_MUX/1 -> MESSAGE_Q_BINARY/1
  MESSAGE_BIT_MUX_COUNTER/1(MESSAGE_BIT_MUX_COUNT) -> Data_IQ_Parser_Counter_Copy/1, Compare To Constant/1, MESSAGE_I_BIT_MUX/1, MESSAGE_Q_BIT_MUX/1
  MESSAGE_I_BIT_MUX/1 -> MESSAGE_I_BINARY/1
  Demux/8 -> MESSAGE_I_BIT_MUX/2
  Demux/7 -> MESSAGE_Q_BIT_MUX/2
  Demux/6 -> MESSAGE_I_BIT_MUX/3
  Demux/5 -> MESSAGE_Q_BIT_MUX/3
  Demux/4 -> MESSAGE_I_BIT_MUX/4
  Demux/3 -> MESSAGE_Q_BIT_MUX/4
  Demux/2 -> MESSAGE_I_BIT_MUX/5
  Demux/1 -> MESSAGE_Q_BIT_MUX/5
  MESSAGE_DATA_BYTE/1 -> Int2Bits/1(u)
  Int2Bits/1(y) -> Demux/1
  Compare To Constant/1 -> Get_New_Data_Byte_For_Mod/1
  INITIALIZE_TX_CORE/1 -> MESSAGE_BIT_MUX_COUNTER/1(INITIALIZE_MESSAGE_BIT_MUX_COUNTER)

== system QPSK_system_v3e/TX_SYSTEM_TOP/TX_CORE_DELAYED_SUBSYSTEM/TX_CORE/GEN_MOD_SHAPED_TX_DATA_PACKET/GEN_MODULATED_TX_DATA_PACKET/Message_Data/QPSK_Modulator ==
  MESSAGE_I_BINARY : Inport
  MESSAGE_Q_BINARY : Inport  Port=2
  Constant1 : Constant  OutDataTypeStr=int8  SampleTime=-1
  Constant2 : Constant  Value=-1  OutDataTypeStr=int8  SampleTime=-1
  Constant3 : Constant  OutDataTypeStr=int8  SampleTime=-1
  Constant4 : Constant  Value=-1  OutDataTypeStr=int8  SampleTime=-1
  MODULATOR_SWITCH_I : Switch  Criteria=u2 ~= 0  RndMeth=Round
  MODULATOR_SWITCH_Q : Switch  Criteria=u2 ~= 0  RndMeth=Round
  MESSAGE_I_MODULATED : Outport
  MESSAGE_Q_MODULATED : Outport  Port=2
  wires:
  MODULATOR_SWITCH_Q/1 -> MESSAGE_Q_MODULATED/1
  Constant4/1 -> MODULATOR_SWITCH_Q/3
  Constant2/1 -> MODULATOR_SWITCH_I/3
  Constant1/1 -> MODULATOR_SWITCH_I/1
  MESSAGE_Q_BINARY/1 -> MODULATOR_SWITCH_Q/2
  Constant3/1 -> MODULATOR_SWITCH_Q/1
  MODULATOR_SWITCH_I/1 -> MESSAGE_I_MODULATED/1
  MESSAGE_I_BINARY/1 -> MODULATOR_SWITCH_I/2

== system QPSK_system_v3e/TX_SYSTEM_TOP/TX_CORE_DELAYED_SUBSYSTEM/TX_CORE/GEN_MOD_SHAPED_TX_DATA_PACKET/GEN_MODULATED_TX_DATA_PACKET/Message_Data/IQ_Parser/MESSAGE_BIT_MUX_COUNTER ==
  INITIALIZE_MESSAGE_BIT_MUX_COUNTER : Inport
  Compare To Constant3 : simulink/Logic and Bit Operations/Compare To Constant  relop=>=  const=4  OutDataTypeStr=boolean  ZeroCross=off
  Constant1 : Constant  OutDataTypeStr=uint32
  Constant2 : Constant  Value=0  OutDataTypeStr=uint32
  Logical Operator : Logic  Operator=OR  AllPortsSameDT=off  OutDataTypeStr=boolean
  Sum : Sum  OutDataTypeStr=uint32  RndMeth=Nearest  SaturateOnIntegerOverflow=on
  Switch1 : Switch  Criteria=u2 ~= 0
  Unit Delay : UnitDelay  SampleTime=-1
  MESSAGE_BIT_MUX_COUNT : Outport
  wires:
  Switch1/1 -> Sum/2, MESSAGE_BIT_MUX_COUNT/1
  Unit Delay/1 -> Compare To Constant3/1, Switch1/3
  Constant2/1 -> Switch1/1
  Sum/1 -> Unit Delay/1
  Constant1/1 -> Sum/1
  Compare To Constant3/1 -> Logical Operator/2
  INITIALIZE_MESSAGE_BIT_MUX_COUNTER/1 -> Logical Operator/1
  Logical Operator/1 -> Switch1/2

== matlab function QPSK_system_v3e/RX_CORE_TOP/RX/rx_double/print/MATLAB Function ==
  data: byte_in input
function  fcn(byte_in)
coder.extrinsic('native2unicode')
persistent index_mess
persistent RecBytes
if isempty(index_mess)
    index_mess = 1;
    RecBytes = zeros(1,18);
end 


RecBytes(index_mess) = byte_in;
index_mess = index_mess+1;

if index_mess == 19
    numRecBytes = RecBytes(1)+RecBytes(2)+RecBytes(3);
    msgBytes = RecBytes((1+4):(numRecBytes+4));
    Message_Received_double = native2unicode(msgBytes)
end

== matlab function QPSK_system_v3e/TX_SYSTEM_TOP/TX_CORE_DELAYED_SUBSYSTEM/TX_CORE/GEN_MOD_SHAPED_TX_DATA_PACKET/GEN_MODULATED_TX_DATA_PACKET/Message_Data/IQ_Parser/Int2Bits ==
  data: u input; y output
function y = fcn(u)
% Converts Integer(8bits) to a 1-D array Bits

y = bitget(u, [8:-1:1])';

== matlab function QPSK_system_v3e/RX_CORE_TOP/RX/dc_offset_fp ==
  data: i_in input; i_out output; q_in input; alpha_in input; gain_en_in input; rssi_low_goal_in input; rssi_high_goal_in input; rx_en_in input; q_out output; rssi_out output; rssi_en_out output; dir_out output; dir_en_out output; d1 output; d2 output; d3 output; d4 output; d5 output; d6 output; d7 output; d8 output; d9 output
function [i_out,q_out,rssi_out,rssi_en_out,dir_out,dir_en_out,d1,d2,d3,d4,d5,d6,d7,d8,d9] = dc_offset_correction_FixPt(i_in,q_in,alpha_in,gain_en_in,rssi_low_goal_in,rssi_high_goal_in,rx_en_in)

fm = hdlfimath;
persistent i_dc q_dc i_mean q_mean
persistent counter rssi_sum
persistent dir_state
persistent rssiHold
persistent noise_offset noise_inc noise_dec
    i_in = fi( i_in, 1, 12, 0, fm );
    q_in = fi( q_in, 1, 12, 0, fm );
    alpha = fi( alpha_in, 0, 12, 0, fm );
    gain_en_in = fi( gain_en_in, 0, 1, 0, fm );
    rssi_low_goal_in = fi( rssi_low_goal_in, 0, 24, 0, fm );
    rssi_high_goal_in = fi( rssi_high_goal_in, 0, 24, 0, fm );
if isempty( i_dc )
    i_dc = fi(0, 1, 24, 12, fm);
    q_dc = fi(0, 1, 24, 12, fm);
    i_mean = fi(0, 1, 24, 12, fm);
    q_mean = fi(0, 1, 24, 12, fm);
    counter = fi(0, 0, 9, 0, fm);
    noise_inc = fi(0, 0, 4, 0, fm);
    noise_dec = fi(0, 0, 2, 0, fm);
    noise_offset = fi(0, 0, 8, 0, fm);
    rssi_sum = fi(0, 0, 32, 0, fm);
    dir_state = fi(0, 0, 1, 0, fm);
    rssiHold = fi(0, 0, 24, 0, fm);
end
%%%%%%%%%%%%%%%%%%%%%%%%%%%%%%%%%%%%%%%%%%%%%%%%%%%%%%%%%%%%%%%%%%%%%%%%%%%
% DC Correction section
%%%%%%%%%%%%%%%%%%%%%%%%%%%%%%%%%%%%%%%%%%%%%%%%%%%%%%%%%%%%%%%%%%%%%%%%%%%
if rx_en_in==1
    i_mean = fi((fi(1, 0, 1, 0) - alpha)*i_mean + alpha*i_in, 1, 24, 12, fm);
    q_mean = fi((fi(1, 0, 1, 0) - alpha)*q_mean + alpha*q_in, 1, 24, 12, fm);
    i_dc = fi((fi(1, 0, 1, 0) - alpha)*i_dc + alpha*i_in, 1, 24, 12, fm);  %update the i dc offset
    q_dc = fi((fi(1, 0, 1, 0) - alpha)*q_dc + alpha*q_in, 1, 24, 12, fm);  %update the q dc offset
    if abs( i_mean )>(fi(50, 0, 6, 0) + noise_offset)  % too much noise, raise cieling.
        noise_inc = fi(noise_inc + fi(1, 0, 1, 0), 0, 4, 0, fm);
        i_dc = fi(0, 1, 24, 12, fm);
    else
        noise_dec = fi(noise_dec + fi(1, 0, 1, 0), 0, 2, 0, fm);
    end
    if abs( q_mean )>(fi(50, 0, 6, 0) + noise_offset)  % too much noise, raise cieling.
        noise_inc = fi(noise_inc + fi(1, 0, 1, 0), 0, 4, 0, fm);
        q_dc = fi(0, 1, 24, 12, fm);
    else
        noise_dec = fi(noise_dec + fi(1, 0, 1, 0), 0, 2, 0, fm);
    end
    if (noise_inc>10)
        %there is a high dc_offset value that needs to be corrected
        noise_offset = fi(noise_offset + fi(10, 0, 4, 0), 0, 8, 0, fm);
        noise_inc = fi(0, 0, 4, 0, fm);
    end
    if (noise_dec>100000)
        %dc offset threshold is higher than needed
        noise_offset = fi(noise_offset - fi(10, 0, 4, 0), 0, 8, 0, fm);
        noise_dec = fi(0, 0, 2, 0, fm);
    end
end
i_out = fi(i_in - i_dc, 1, 12, 0, fm);
q_out = fi(q_in - q_dc, 1, 12, 0, fm);
%correct false positive/nagatives
if (abs( i_mean )<50)
    noise_inc = fi(0, 0, 4, 0, fm);
end
if (abs( i_mean )>noise_offset - fi(10, 0, 4, 0))
    noise_dec = fi(0, 0, 2, 0, fm);
end
%%%%%%%%%%%%%%%%%%%%%%%%%%%%%%%%%%%%%%%%%%%%%%%%%%%%%%%%%%%%%%%%%%%%%%%%%%%
%%%%%%%%%%%%%%%%%%%%%%%%%%%%%%%%%%%%%%%%%%%%%%%%%%%%%%%%%%%%%%%%%%%%%%%%%%%
% RSSI Estimation
%%%%%%%%%%%%%%%%%%%%%%%%%%%%%%%%%%%%%%%%%%%%%%%%%%%%%%%%%%%%%%%%%%%%%%%%%%%
rssi_inst = fi(i_out*i_out + q_out*q_out, 0, 23, 0, fm);
rssi_en_out = fi(0, 0, 1, 0, fm);
rssi_out = fi(0, 0, 24, 0, fm);
if rx_en_in==1
    if counter==0 && rssi_inst>fi(2, 0, 2, 0)*fi(50, 0, 6, 0)*fi(50, 0, 6, 0)
        counter = fi(1, 0, 9, 0, fm);
        rssi_sum = fi(0, 0, 32, 0, fm);
    end
    if counter~=0
        if rssi_inst<fi(2, 0, 2, 0)*fi(50, 0, 6, 0)*fi(50, 0, 6, 0)
            counter = fi(0, 0, 9, 0, fm);
        else
            counter = fi(counter + fi(1, 0, 1, 0), 0, 9, 0, fm);
            rssi_sum = fi(rssi_sum + rssi_inst, 0, 32, 0, fm);
            if counter>=2^8
                counter = fi(0, 0, 9, 0, fm);
                rssi_out = fi(round( fi_div_by_shift(rssi_sum, 8) ), 0, 24, 0, fm);
                rssiHold = fi(rssi_out, 0, 24, 0, fm);
                rssi_en_out = fi(1, 0, 1, 0, fm);
            end
        end
    end
end
%%%%%%%%%%%%%%%%%%%%%%%%%%%%%%%%%%%%%%%%%%%%%%%%%%%%%%%%%%%%%%%%%%%%%%%%%%%
%%%%%%%%%%%%%%%%%%%%%%%%%%%%%%%%%%%%%%%%%%%%%%%%%%%%%%%%%%%%%%%%%%%%%%%%%%%
% Gain Correction
%%%%%%%%%%%%%%%%%%%%%%%%%%%%%%%%%%%%%%%%%%%%%%%%%%%%%%%%%%%%%%%%%%%%%%%%%%%
dir_out = fi(0, 0, 2, 0, fm);
dir_en_out = fi(0, 0, 1, 0, fm);
% dir_out = 0 - do nothing
% dir_out = 1 - increase
% dir_out = 2 - decrease
ai = fi(abs( i_in ), 0, 11, 0, fm);
aq = fi(abs( q_in ), 0, 11, 0, fm);
% only increase power if the rssi is away from the mean
rssi_diff = fi(abs( rssiHold - (i_mean*i_mean + q_mean*q_mean) ), 0, 24, 0, fm);
if rx_en_in==1
    switch fi_toint(dir_state)
        case 0  % wait for some action and the processor is done
            if gain_en_in==0
                if rssi_en_out==1
                    if rssi_diff<rssi_low_goal_in  %too low - increase
                        dir_out = fi(1, 0, 2, 0, fm);
                        dir_en_out = fi(1, 0, 1, 0, fm);
                        dir_state = fi(1, 0, 1, 0, fm);
                    end
                    if rssi_diff>rssi_high_goal_in  %too high - decrease
                        dir_out = fi(2, 0, 2, 0, fm);
                        dir_en_out = fi(1, 0, 1, 0, fm);
                        dir_state = fi(1, 0, 1, 0, fm);
                    end
                end
                % we're saturating the ADC so decrease gain
                % this overrides anything else
                if (ai>1500) || (aq>1500)
                    dir_out = fi(2, 0, 2, 0, fm);  % decrease
                    dir_en_out = fi(1, 0, 1, 0, fm);
                    dir_state = fi(1, 0, 1, 0, fm);
                end
            end
        case 1  % see if the MCU has done something and if so reset
            if gain_en_in==1
                dir_out = fi(0, 0, 2, 0, fm);
                dir_en_out = fi(1, 0, 1, 0, fm);
                dir_state = fi(0, 0, 1, 0, fm);
            end
        otherwise
            dir_state = fi(0, 0, 1, 0, fm);
    end
end
d1 = fi(i_in, 1, 12, 0, fm);
d2 = fi(i_mean, 1, 12, 0, fm);
d3 = fi(i_dc, 1, 12, 0, fm);
d4 = fi(rssiHold, 0, 24, 0, fm);
d5 = fi(rssi_diff, 0, 24, 0, fm);
d6 = fi(dir_state, 0, 1, 0, fm);
d7 = fi(gain_en_in, 0, 1, 0, fm);
d8 = fi(dir_out, 0, 2, 0, fm);
d9 = fi(dir_en_out, 0, 1, 0, fm);
%%%%%%%%%%%%%%%%%%%%%%%%%%%%%%%%%%%%%%%%%%%%%%%%%%%%%%%%%%%%%%%%%%%%%%%%%%%
end


function y = fi_div_by_shift(a,shift_len)
coder.inline( 'always' );
if isfi( a )
    nt = numerictype( a );
    fm = fimath( a );
    nt_bs = numerictype( nt.Signed, nt.WordLength + shift_len, nt.FractionLength + shift_len );
    y = bitsrl( fi( a, nt_bs, fm ), shift_len );
else
    y = a/2^shift_len;
end
end


function y = fi_toint(u)
coder.inline( 'always' );
if isfi( u )
    nt = numerictype( u );
    s = nt.SignednessBool;
    wl = nt.WordLength;
    y = int32( fi( u, s, wl, 0, hdlfimath ) );
else
    y = int32( u );
end
end
